simulink model "FullAdder"  (R2014a)
settings: Solver=ode45  StartTime=0.0  StopTime=inf  RelTol=1e-3
settings Model: Creator=nunkesser  LastModifiedBy=nunkesser

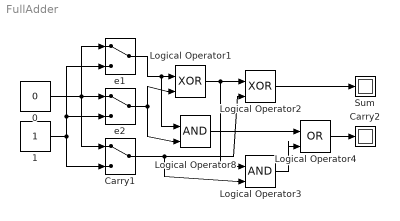
== system FullAdder ==
  0 : Constant  Value=0  OutDataTypeStr=boolean
  1 : Constant  OutDataTypeStr=boolean
  Carry1 : ManualSwitch
  Carry2 : Display
  Logical Operator1 : Logic  Operator=XOR  IconShape=distinctive  AllPortsSameDT=off  OutDataTypeStr=boolean
  Logical Operator2 : Logic  Operator=XOR  IconShape=distinctive  AllPortsSameDT=off  OutDataTypeStr=boolean
  Logical Operator3 : Logic  IconShape=distinctive  AllPortsSameDT=off  OutDataTypeStr=boolean
  Logical Operator4 : Logic  Operator=OR  IconShape=distinctive  AllPortsSameDT=off  OutDataTypeStr=boolean
  Logical Operator8 : Logic  IconShape=distinctive  AllPortsSameDT=off  OutDataTypeStr=boolean
  Sum : Display
  e1 : ManualSwitch
  e2 : ManualSwitch
  wires:
  0/1 -> e1/1, Carry1/1, e2/1
  1/1 -> Carry1/2, e2/2, e1/2
  e1/1 -> Logical Operator8/1, Logical Operator1/1
  e2/1 -> Logical Operator8/2, Logical Operator1/2
  Logical Operator1/1 -> Logical Operator2/1, Logical Operator3/1
  Carry1/1 -> Logical Operator3/2, Logical Operator2/2
  Logical Operator2/1 -> Sum/1
  Logical Operator8/1 -> Logical Operator4/1
  Logical Operator3/1 -> Logical Operator4/2
  Logical Operator4/1 -> Carry2/1
